simulink model "Motor"  (R2018b)
settings: Solver=FixedStepAuto  StartTime=0.0  StopTime=10  FixedStep=0.001  RelTol=1e-3
settings Model: Creator=chengqian  LastModifiedBy=chengqian

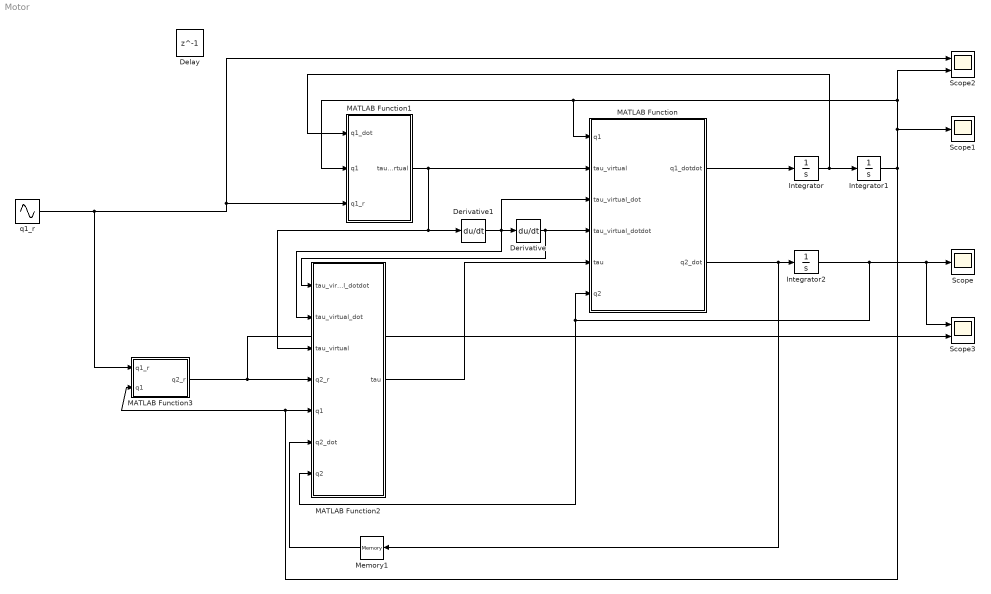
== system Motor ==
  Delay : Delay  DelayLength=1  InitialCondition=0
  Derivative : Derivative
  Derivative1 : Derivative
  Integrator : Integrator
  Integrator1 : Integrator
  Integrator2 : Integrator
  MATLAB Function : MATLAB Function  TreatAsAtomicUnit=on
  MATLAB Function1 : MATLAB Function  TreatAsAtomicUnit=on
  MATLAB Function2 : MATLAB Function  TreatAsAtomicUnit=on
  MATLAB Function3 : MATLAB Function  TreatAsAtomicUnit=on
  Memory1 : Memory
  Scope : Scope
  Scope1 : Scope
  Scope2 : Scope  NumInputPorts=2
  Scope3 : Scope  NumInputPorts=2
  q1_r : Sin  SampleTime=0
  wires:
  Derivative/1 -> MATLAB Function/4(tau_virtual_dotdot), MATLAB Function2/1(tau_virtual_dotdot)
  Derivative1/1 -> MATLAB Function/3(tau_virtual_dot), Derivative/1, MATLAB Function2/2(tau_virtual_dot)
  MATLAB Function1/1(tau_virtual) -> Derivative1/1, MATLAB Function2/3(tau_virtual), MATLAB Function/2(tau_virtual)
  MATLAB Function2/1(tau) -> MATLAB Function/5(tau)
  q1_r/1 -> MATLAB Function3/1(q1_r), Scope2/1, MATLAB Function1/3(q1_r)
  MATLAB Function3/1(q2_r) -> Scope3/2, MATLAB Function2/4(q2_r)
  Integrator/1 -> MATLAB Function1/1(q1_dot), Integrator1/1
  Integrator1/1 -> MATLAB Function3/2(q1), MATLAB Function2/5(q1), Scope2/2, MATLAB Function/1(q1), MATLAB Function1/2(q1), Scope1/1
  Integrator2/1 -> MATLAB Function2/7(q2), MATLAB Function/6(q2), Scope3/1, Scope/1
  MATLAB Function/2(q2_dot) -> Integrator2/1, Memory1/1
  MATLAB Function/1(q1_dotdot) -> Integrator/1
  Memory1/1 -> MATLAB Function2/6(q2_dot)

== matlab function Motor/MATLAB Function1 ==
  data: q1_dot input; tau_virtual output; q1 input; q1_r input
function tau_virtual = fcn(q1_dot,q1,q1_r)

T = 10;
J = 0.0101;
M = 0.0320;
K = 4000;

beta1 = 2; beta2 = 2;
alpha1 = 10; alpha2 = 10;
Kp1 = 100; Kd1 =20;

rol1 = norm((-T - K*q1 + M*q1_dot));
e1 = q1_r - q1;
tau_virtual = e1 + (1/K)*((-alpha1*rol1^2-beta1)*(q1+q1_dot) + (-Kp1*q1-Kd1*q1_dot));

== matlab function Motor/MATLAB Function ==
  data: q1 input; tau_virtual input; tau_virtual_dot input; tau_virtual_dotdot input; tau input; q1_dotdot output; q2 input; q2_dot output
function [q1_dotdot,q2_dot] = fcn(q1,tau_virtual,tau_virtual_dot,tau_virtual_dotdot,tau,q2)

T = 10;
J = 0.0101;
M = 0.0320;
K = 4000;

beta1 = 2; beta2 = 2;
alpha1 = 10; alpha2 = 10;
Kp1 = 100; Kd1 =20;



q1_dotdot = (- T - K*q1 + K*(q2 - tau_virtual) + K*tau_virtual)/M;
q2_dot = (-J*tau_virtual_dotdot + K*q1 - K*(q2 - tau_virtual) - K*tau_virtual + tau)/J + tau_virtual_dot;

== matlab function Motor/MATLAB Function2 ==
  data: tau_virtual_dotdot input; tau_virtual_dot input; tau_virtual input; q2_r input; tau output; q1 input; q2_dot input; q2 input
function tau = fcn(tau_virtual_dotdot,tau_virtual_dot,tau_virtual,q2_r,q1,q2_dot,q2)

T = 10;
J = 0.0101;
M = 0.0320;
K = 4000;

beta1 = 2; beta2 = 2;
alpha1 = 10; alpha2 = 10;
Kp1 = 100; Kd1 =20;

rol2 = norm((-J*tau_virtual_dotdot - K*(q2-tau_virtual) + K*q1 - K*tau_virtual + J*(q2_dot-tau_virtual_dot)));
e2 = q2_r - q2;
tau = e2 + (-alpha2*rol2^2- beta2)*(q2_dot-tau_virtual_dot + q2-tau_virtual);

== matlab function Motor/MATLAB Function3 ==
  data: q1_r input; q2_r output; q1 input
function q2_r = fcn(q1_r,q1)

T = 10;
J = 0.0101;
M = 0.0320;
K = 4000;

beta1 = 2; beta2 = 2;
alpha1 = 10; alpha2 = 10;
Kp1 = 100; Kd1 =20;

q2_r = (-M*q1_r + T + K*q1)/K;
